simulink model "Discrete_FOC_LSM_v1_v25b"  (R2025b)
settings: Solver=FixedStepAuto  StopTime=4  FixedStep=1e-4  MaxStep=0.001
values from neighbouring files (symbols this model uses):
  airgap_vec = 14.5:1:16.5    [CargarDatosModeloLSM.m]
  Distance_between_EMS = 0.768    [CargarDatosModeloLSM.m]
  force_drag_vec = []    [CargarDatosModeloLSM.m]
  hems_n = 4    [CargarDatosModeloLSM.m]
  initial_angle = 0.63    [CargarDatosModeloLSM.m]
  kd = 0.0518    [CargarDatosModeloLSM.m]
  mass = 250    [CargarDatosModeloLSM.m]
  max_voltage = 300    [CargarDatosModeloLSM.m]
  real_airgap = 14.5    [CargarDatosModeloLSM.m]
  speed_drag_vec = 0:5:60    [CargarDatosModeloLSM.m]
  speed_reference_ms = speed_reference/3.6    (= 6.94444444444)    [CargarDatosModeloLSM.m]
  speetec_end = 4 + 2*Distance_between_EMS + 0.5    (= 6.036)    [CargarDatosModeloLSM.m]
  speetec_init = 1 - 0.0925    (= 0.9075)    [CargarDatosModeloLSM.m]
  speetec_offset = 0.174 + 0.116 + 0.0925    (= 0.3825)    [CargarDatosModeloLSM.m]
undefined symbols (not defined in the file or in its folder): angulos, frac_polar, fuerza, magnitude, Resistencia
libraries: slpidlib x3
(part 2 of 2)

== matlab function Discrete_FOC_LSM_v1_v25b/LSM model/Sensor de Corriente/Sensor corriente V/Discretizado Amplitud ==
  data: valor input; valor_discretizado output; num_valores input; max input; min input
function valor_discretizado = fcn(valor, num_valores, max, min)

if valor > max
    valor_discretizado = max;
    return
end

if valor < min
    valor_discretizado = min;
    return
end


valor_escalon = (max - min)/(num_valores - 1);


i = min;


while (i < max)
    if (i + valor_escalon/2 > valor)
        valor_discretizado = i;
        return
    end

    i = i + valor_escalon;
end


valor_discretizado = max;

end

== matlab function Discrete_FOC_LSM_v1_v25b/LSM model/Sensor de Corriente/Sensor corriente V/MATLAB Function1 ==
  data: V input; I output
function I = fcn(V)

I = (V - 2.5)/0.005;
